simulink model "LQR_Regler_V1"  (R2019b)
settings: Solver=VariableStepAuto  StartTime=0.0  StopTime=100  RelTol=1e-3
values from neighbouring files (symbols this model uses):
  A = [a Znm; -c Zmm]    [LQG_example.m]    (also in Linearize.m = double(subs(A_mat,[alpha,beta,gamma,F_f,F_b],[x_s(1:3),u_s(1)
  B = [b;-d]    [LQG_example.m]    (also in Linearize.m = double(subs(B_mat,[alpha,beta,gamma],x_s(1:3))))
  C = [eye(3),zeros(3,3)]    [Linearize.m]
  D = zeros(3,2)    [Linearize.m]
  L = L'    [LQR_controller.m]
  u_s = zeros(2,1)    [Linearize.m]
  Vorfilter = -inv(C_LQI*inv(A-B*K_LQR)*B)    [LQR_controller.m]
undefined symbols (not defined in the file or in its folder): K_LQI
libraries: simulink x6
settings Model: Creator=qinjiaqi  LastModifiedBy=qinjiaqi

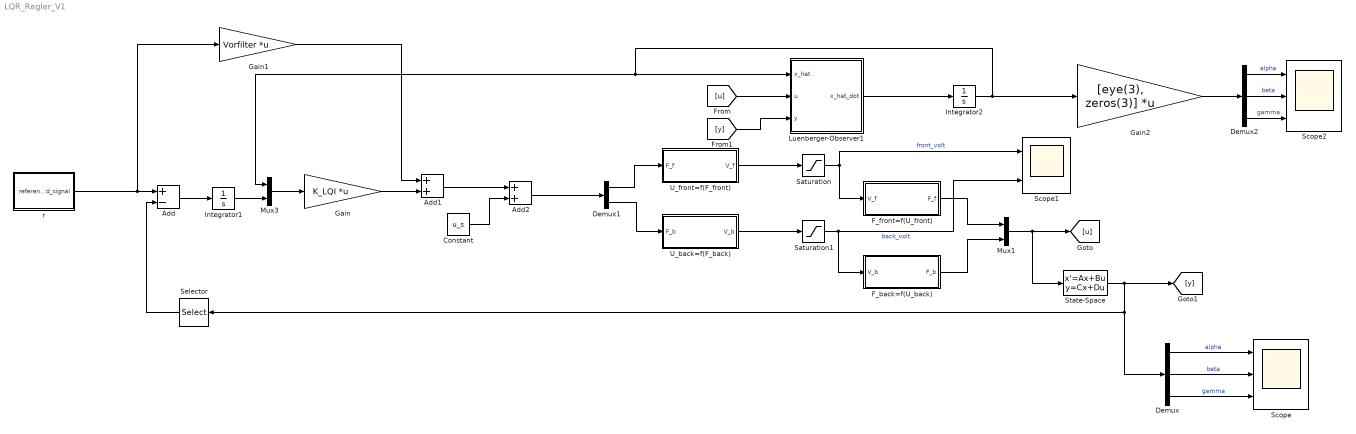
== system LQR_Regler_V1 ==
  Add : Sum  Inputs=+-
  Add1 : Sum
  Add2 : Sum
  Constant : Constant  Value=u_s
  Demux : Demux  Outputs=3
  Demux1 : Demux  Outputs=2
  Demux2 : Demux  Outputs=3
  F_back=f(U_back) : Subsystem
  F_front=f(U_front) : Subsystem
  Gain : Gain  Gain=K_LQI  Multiplication=Matrix(K*u) (u vector)
  Gain1 : Gain  Gain=Vorfilter  Multiplication=Matrix(K*u) (u vector)
  Gain2 : Gain  Gain=[eye(3), zeros(3)]  Multiplication=Matrix(K*u) (u vector)
  Integrator1 : Integrator
  Integrator2 : Integrator
  Luenberger-Observer1 : MATLAB Function  TreatAsAtomicUnit=on
  Mux1 : Mux  Inputs=2
  Mux3 : Mux  Inputs=2
  Saturation : Saturate  UpperLimit=4  LowerLimit=0
  Saturation1 : Saturate  UpperLimit=4  LowerLimit=0
  Scope : Scope  NumInputPorts=3
  Scope1 : Scope  NumInputPorts=2
  Scope2 : Scope  NumInputPorts=3
  Selector : Selector  InputPortWidth=3  IndexOptions=Index vector (dialog)  Indices=[1 2]  OutputSizes=1
  State-Space : StateSpace  A=A  B=B  C=C  D=D  InitialCondition=0
  U_back=f(F_back) : Subsystem
  U_front=f(F_front) : Subsystem
  "r " : Subsystem
  wires:
  Add/1 -> Integrator1/1
  "r "/1(referenced_signal) -> Gain1/1, Add/1
  Integrator1/1 -> Mux3/2
  Mux3/1 -> Gain/1
  Gain/1 -> Add1/2
  Luenberger-Observer1/1(x_hat_dot) -> Integrator2/1
  Integrator2/1 -> Mux3/1, Luenberger-Observer1/1(x_hat), Gain2/1
  Gain1/1 -> Add1/1
  Selector/1 -> Add/2
  Demux/1 -> Scope/1  "alpha"
  Demux/2 -> Scope/2  "beta"
  Demux/3 -> Scope/3  "gamma"
  Add1/1 -> Add2/1
  Constant/1 -> Add2/2
  Add2/1 -> Demux1/1
  Demux1/1 -> U_front=f(F_front)/1(F_f)
  Demux1/2 -> U_back=f(F_back)/1(F_b)
  U_front=f(F_front)/1(V_f) -> Saturation/1
  U_back=f(F_back)/1("V_b ") -> Saturation1/1
  Saturation/1 -> F_front=f(U_front)/1(V_f), Scope1/1  "front_volt"
  Saturation1/1 -> Scope1/2, F_back=f(U_back)/1(V_b)  "back_volt"
  F_front=f(U_front)/1(F_f) -> Mux1/1
  F_back=f(U_back)/1(F_b) -> Mux1/2
  Mux1/1 -> State-Space/1, [u]
  [u] -> Luenberger-Observer1/2(u)
  State-Space/1 -> Selector/1, Demux/1, [y]
  [y] -> Luenberger-Observer1/3(y)
  Gain2/1 -> Demux2/1
  Demux2/1 -> Scope2/1  "alpha"
  Demux2/2 -> Scope2/2  "beta"
  Demux2/3 -> Scope2/3  "gamma"

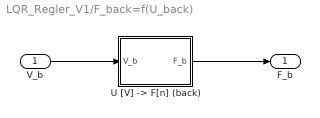
== system LQR_Regler_V1/F_back=f(U_back) ==
  V_b : Inport
  "U [V] -> F[n] (back)" : MATLAB Function  TreatAsAtomicUnit=on
  F_b : Outport
  wires:
  "U [V] -> F[n] (back)"/1(F_b) -> F_b/1
  V_b/1 -> "U [V] -> F[n] (back)"/1(V_b)

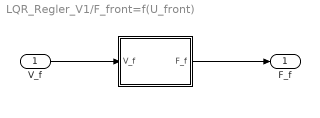
== system LQR_Regler_V1/F_front=f(U_front) ==
  V_f : Inport
  " " : MATLAB Function  TreatAsAtomicUnit=on
  F_f : Outport
  wires:
  V_f/1 -> " "/1(V_f)
  " "/1(F_f) -> F_f/1

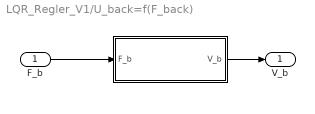
== system LQR_Regler_V1/U_back=f(F_back) ==
  F_b : Inport
  " " : MATLAB Function  TreatAsAtomicUnit=on
  "V_b " : Outport
  wires:
  F_b/1 -> " "/1(F_b)
  " "/1(V_b) -> "V_b "/1

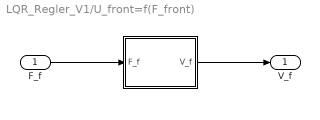
== system LQR_Regler_V1/U_front=f(F_front) ==
  F_f : Inport
  " " : MATLAB Function  TreatAsAtomicUnit=on
  V_f : Outport
  wires:
  " "/1(V_f) -> V_f/1
  F_f/1 -> " "/1(F_f)

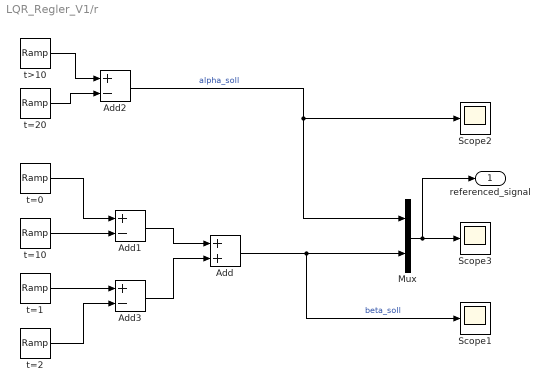
== system LQR_Regler_V1/r  ==
  Add : Sum
  Add1 : Sum  Inputs=+-
  Add2 : Sum  Inputs=+-
  Add3 : Sum  Inputs=+-
  Mux : Mux  Inputs=2
  Scope1 : Scope
  Scope2 : Scope
  Scope3 : Scope
  t=0 : simulink/Sources/Ramp  slope=27*pi/(5*180)  start=0  InitialOutput=-27*pi/180
  t=1 : simulink/Sources/Ramp  slope=-27*pi/(5*180)  start=18  InitialOutput=0
  t=10 : simulink/Sources/Ramp  slope=27*pi/(5*180)  start=5  InitialOutput=0
  t=2 : simulink/Sources/Ramp  slope=-27*pi/(5*180)  start=23  InitialOutput=0
  t=20 : simulink/Sources/Ramp  slope=90*pi/(5*180)  start=15  InitialOutput=0
  t>10 : simulink/Sources/Ramp  slope=90*pi/(5*180)  start=10  InitialOutput=0
  referenced_signal : Outport
  wires:
  Mux/1 -> referenced_signal/1, Scope3/1
  t=20/1 -> Add2/2
  t=10/1 -> Add1/2
  t>10/1 -> Add2/1
  Add2/1 -> Mux/1, Scope2/1  "alpha_soll"
  t=0/1 -> Add1/1
  Add1/1 -> Add/1
  Add/1 -> Mux/2, Scope1/1  "beta_soll"
  t=1/1 -> Add3/1
  t=2/1 -> Add3/2
  Add3/1 -> Add/2

== matlab function LQR_Regler_V1/Luenberger-Observer1 ==
  data: x_hat input; u input; x_hat_dot output; y input; A parameter; B parameter; C parameter; L parameter
function x_hat_dot  = fcn(x_hat,u,y,A, B, C, L)
%   x_hat_dot = A*x_hat + B*u + L*(y-y_hat);
%   y_hat = C*x_hat;
    x_hat_dot = (A-L*C)*x_hat + B*u + L*y;

end

== matlab function LQR_Regler_V1/F_back=f(U_back)/U [V] -> F[n] (back) ==
  data: V_b input; F_b output
function F_b = fcn(V_b)

    F_b=0.0462*V_b^2; 
end

== matlab function LQR_Regler_V1/F_front=f(U_front)/  ==
  data: V_f input; F_f output
function F_f = fcn(V_f)

    F_f = 0.0604*V_f^2; 
end

== matlab function LQR_Regler_V1/U_front=f(F_front)/  ==
  data: F_f input; V_f output
function V_f = fcn(F_f)

if F_f<0
    V_f = -(abs(F_f/0.0604)^(1/2));
else
    V_f = (abs(F_f/0.0604)^(1/2));
end

== matlab function LQR_Regler_V1/U_back=f(F_back)/  ==
  data: F_b input; V_b output
function V_b = fcn(F_b)

if F_b<0
    V_b = -(abs(F_b/0.0604)^(1/2));
else
    V_b = (abs(F_b/0.0604)^(1/2));
end
